simulink model "sphere_6SUR_mech"  (R2017a)
settings: Solver=FixedStepAuto  StartTime=0.0  StopTime=100  FixedStep=0.001  RelTol=1e-2  EnableMultiTasking=on
undefined symbols (not defined in the file): m, rad, s
libraries: mblibv1 x69, simulink x3, instrumentlib x1
(part 1 of 2)
settings Model: SimulationMode=accelerator  Creator=ivanp7  LastModifiedBy=ivanp7
settings OptimizationCC: LifeSpan=inf
settings DebuggingCC: AlgebraicLoopMsg=none  SFUnexpectedBacktrackingDiag=warning  SFNoUnconditionalDefaultTransitionDiag=warning  SFExecutionAtInitializationDiag=none
settings GRTTargetCC: TargetLangStandard=C89/C90 (ANSI)  GeneratePreprocessorConditionals=Disable all
settings ConfigComp: CovMetricSettings=dw  CovHtmlReporting=on  CovSaveCumulativeToWorkspaceVar=on  CovSaveSingleToWorkspaceVar=on  CovExternalEMLEnable=off
settings SimMechanicsCC: LastVizWinPosition=[1141 536 560 420]  CamPosition=[4.37083;-0.373326;26.621;]  CamTarget=[4.37083;-0.373326;0;]  CamUpVector=[0;1;0;]  CamHeight=73.1719  VisBackgroundColor=[0.9;0.9;0.95;]  DefaultBodyColor=[1;0;0;]

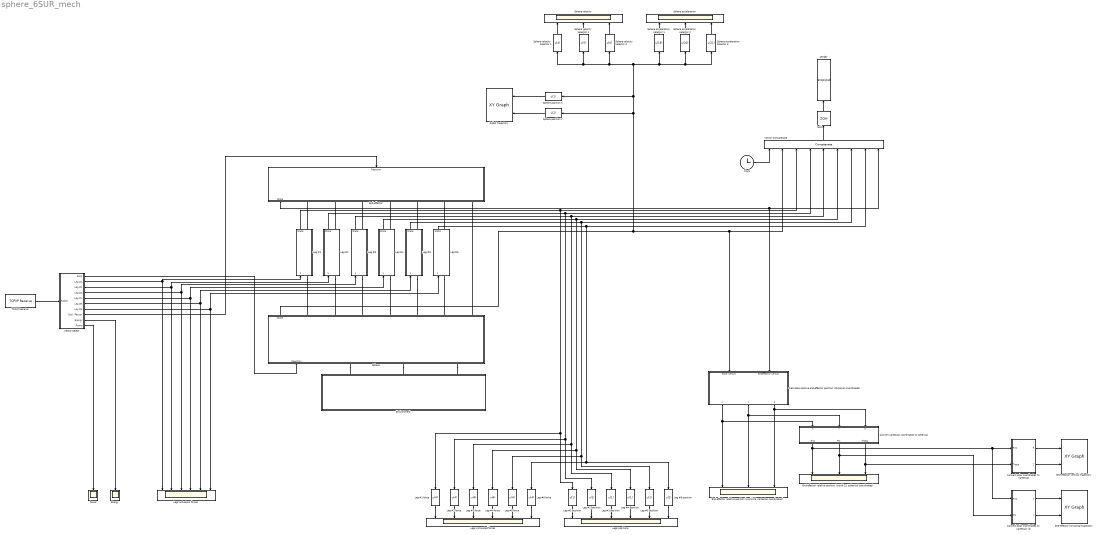
== system sphere_6SUR_mech ==
  Calculate relative end-effector position (cartesian coordinates) : Subsystem
  Convert cartesian coordinates to spherical : Subsystem
  Convert polar coordinates to cartesian : Subsystem
  Convert polar coordinates to cartesian (2) : Subsystem
  End-effector : Subsystem  mask{endeffector_radius=0.25, endeffector_mass=1, endeffector_inertia_coef=2/5}
      mask prompts: endeffector_radius "End-effector radius, m"; endeffector_mass "End-effector mass, kg"; endeffector_inertia_coef "End-effector inertia coefficient"
  End-effector horizontal trajectory : simulink/Sinks/XY Graph  xmin=-1  xmax=1  ymin=-1  ymax=1  st=-1
  "End-effector relative position (world CS, cartesian coordinates)" : Scope  NumInputPorts=3
  "End-effector relative position (world CS, spherical coordinates)" : Scope  NumInputPorts=3
  End-effector vertical trajectory : simulink/Sinks/XY Graph  xmin=0  xmax=1  ymin=-1  ymax=1  st=-1
  Energy : Scope
  Environment : Subsystem  mask{sphere_radius=1, initial_velocity_x=0, initial_velocity_y=0}
      mask prompts: sphere_radius "Sphere radius, m"; initial_velocity_x "Initial velocity (x-axis), m/s"; initial_velocity_y "Initial velocity (y-axis), m/s"
  Leg #1 : Subsystem  mask{ru_mass=0.005, us_mass=0.005, r_axis=[0.505879 -0.310617 0.804738], u_axis1=[0.505879 -0.310617 0.804738], u_axis2=[0.533176 -0.620769 -0.574777], r_coord=[0.12647 -0.0776543 0.201184], u_coord=[-0.382099 -0.61753 0.3125], s_coord=[0 0 1]}
      mask prompts: ru_mass "R-U chain mass, kg"; us_mass "U-S chain mass, kg"; r_axis "R joint axis"; u_axis1 "U joint axis 1"; u_axis2 "U joint axis 2"; r_coord "R joint coordinates"; u_coord "U joint coordinates"; s_coord "S joint coordinates"
  Leg #1 force : Fcn  Expr=u(4)
  Leg #1 position : Fcn  Expr=u(1)
  Leg #2 : Subsystem  mask{ru_mass=0.005, us_mass=0.005, r_axis=[-0.505879 0.310617 -0.804738], u_axis1=[-0.505879 0.310617 -0.804738], u_axis2=[-0.533176 0.620769 0.574777], r_coord=[-0.12647 0.0776543 -0.201184], u_coord=[0.382099 0.61753 -0.3125], s_coord=[0 0 -1]}
      mask prompts: ru_mass "R-U chain mass, kg"; us_mass "U-S chain mass, kg"; r_axis "R joint axis"; u_axis1 "U joint axis 1"; u_axis2 "U joint axis 2"; r_coord "R joint coordinates"; u_coord "U joint coordinates"; s_coord "S joint coordinates"
  Leg #2 force : Fcn  Expr=u(4)
  Leg #2 position : Fcn  Expr=u(1)
  Leg #3 : Subsystem  mask{ru_mass=0.005, us_mass=0.005, r_axis=[0.804738 0.505879 -0.310617], u_axis1=[0.804738 0.505879 -0.310617], u_axis2=[-0.574777 0.533176 -0.620769], r_coord=[0.201184 0.12647 -0.0776543], u_coord=[0.3125 -0.382099 -0.61753], s_coord=[1 0 0]}
      mask prompts: ru_mass "R-U chain mass, kg"; us_mass "U-S chain mass, kg"; r_axis "R joint axis"; u_axis1 "U joint axis 1"; u_axis2 "U joint axis 2"; r_coord "R joint coordinates"; u_coord "U joint coordinates"; s_coord "S joint coordinates"
  Leg #3 force : Fcn  Expr=u(4)
  Leg #3 position : Fcn  Expr=u(1)
  Leg #4 : Subsystem  mask{ru_mass=0.005, us_mass=0.005, r_axis=[-0.804738 -0.505879 0.310617], u_axis1=[-0.804738 -0.505879 0.310617], u_axis2=[0.574777 -0.533176 0.620769], r_coord=[-0.201184 -0.12647 0.0776543], u_coord=[-0.3125 0.382099 0.61753], s_coord=[-1 0 0]}
      mask prompts: ru_mass "R-U chain mass, kg"; us_mass "U-S chain mass, kg"; r_axis "R joint axis"; u_axis1 "U joint axis 1"; u_axis2 "U joint axis 2"; r_coord "R joint coordinates"; u_coord "U joint coordinates"; s_coord "S joint coordinates"
  Leg #4 force : Fcn  Expr=u(4)
  Leg #4 position : Fcn  Expr=u(1)
  Leg #5 : Subsystem  mask{ru_mass=0.005, us_mass=0.005, r_axis=[-0.310617 0.804738 0.505879], u_axis1=[-0.310617 0.804738 0.505879], u_axis2=[-0.620769 -0.574777 0.533176], r_coord=[-0.0776543 0.201184 0.12647], u_coord=[-0.61753 0.3125 -0.382099], s_coord=[0 1 0]}
      mask prompts: ru_mass "R-U chain mass, kg"; us_mass "U-S chain mass, kg"; r_axis "R joint axis"; u_axis1 "U joint axis 1"; u_axis2 "U joint axis 2"; r_coord "R joint coordinates"; u_coord "U joint coordinates"; s_coord "S joint coordinates"
  Leg #5 force : Fcn  Expr=u(4)
  Leg #5 position : Fcn  Expr=u(1)
  Leg #6 : Subsystem  mask{ru_mass=0.005, us_mass=0.005, r_axis=[0.310617 -0.804738 -0.505879], u_axis1=[0.310617 -0.804738 -0.505879], u_axis2=[0.620769 0.574777 -0.533176], r_coord=[0.0776543 -0.201184 -0.12647], u_coord=[0.61753 -0.3125 0.382099], s_coord=[0 -1 0]}
      mask prompts: ru_mass "R-U chain mass, kg"; us_mass "U-S chain mass, kg"; r_axis "R joint axis"; u_axis1 "U joint axis 1"; u_axis2 "U joint axis 2"; r_coord "R joint coordinates"; u_coord "U joint coordinates"; s_coord "S joint coordinates"
  Leg #6 force : Fcn  Expr=u(4)
  Leg #6 position : Fcn  Expr=u(1)
  Legs actuators forces : Scope  NumInputPorts=6
  Legs computed forces : Scope  NumInputPorts=6
  Legs positions : Scope  NumInputPorts=6
  Power : Scope
  Robot trajectory : simulink/Sinks/XY Graph  xmin=-100  xmax=100  ymin=-100  ymax=100  st=-1
  Sphere : Subsystem  mask{sphere_radius=1, sphere_mass=0.1, sphere_inertia_coef=2/3}
      mask prompts: sphere_radius "Sphere radius, m"; sphere_mass "Sphere mass, kg"; sphere_inertia_coef "Sphere inertia coefficient, m"
  Sphere acceleration selector 1 : Fcn  Expr=u(19)
  Sphere acceleration selector 2 : Fcn  Expr=u(20)
  Sphere acceleration selector 3 : Fcn  Expr=u(21)
  Sphere velocity selector 1 : Fcn  Expr=u(4)
  Sphere velocity selector 2 : Fcn  Expr=u(5)
  Sphere velocity selector 3 : Fcn  Expr=u(6)
  Sphere acceleration : Scope  NumInputPorts=3
  Sphere position X : Fcn  Expr=u(1)
  Sphere position Y : Fcn  Expr=u(2)
  Sphere velocity : Scope  NumInputPorts=3
  TCP/IP Receive : instrumentlib/TCP//IP Receive  Priority=1  Host=localhost  Port=61111  DataSize="[1  20]"  EnableBlockingMode=on  Timeout=1  SampleTime=0.001  DataType=double  ByteOrder=LittleEndian
      settings: SourceProductName=Instrument Control Toolbox
  Vector Concatenate : Concatenate  NumInputs=9
  Vector Select : Subsystem
  clock : Clock
      settings: Decimation=1000
  hold : ZeroOrderHold  SampleTime=-1
  sender : M-S-Function  Priority=2  DialogController=instrumentcreatedialog  FunctionName=stcpipsb  Parameters=Host, Port, EnableBlockingMode, Timeout, ByteOrder  DisplayMFileStacktrace=off  mask(TCP/IP Send){Host=localhost, Port=61112, EnableBlockingMode=on, Timeout=1, ByteOrder=LittleEndian}
      mask prompts: Port "Remote Port:"; EnableBlockingMode "Enable blocking mode"; ByteOrder "Byte order:"
      mask help: Send data over TCP/IP network to a specified remote machine.
      mask init:
      | [str port] = instrumentslgate('privateslgetdisplaystring', EnableBlockingMode);
      mask Help: eval('helpview(fullfile(docroot, ''toolbox'', ''instrument'', ''instrument.map''), ''ICT_tcpipsend_Block'')');
      mask TypeOptions ByteOrder: BigEndian | LittleEndian
      mask Display:
      | disp(str);
      | port_label('input',port(1).id,port(1).label);
  wires:
  Leg #1/1(State) -> Vector Concatenate/3, Leg #1 force/1, Leg #1 position/1
  Leg #2/1(State) -> Leg #2 force/1, Leg #2 position/1, Vector Concatenate/4
  Leg #3/1(State) -> Vector Concatenate/5, Leg #3 force/1, Leg #3 position/1
  End-effector/1(State) -> Calculate relative end-effector position (cartesian coordinates)/2(Endeffector sensor), Vector Concatenate/9
  Leg #1 position/1 -> Legs positions/1
  Leg #2 position/1 -> Legs positions/2
  Leg #3 position/1 -> Legs positions/3
  Vector Select/4(Leg #3) -> Leg #3/1(Reaction), Legs actuators forces/3
  Vector Select/2(Leg #1) -> Legs actuators forces/1, Leg #1/1(Reaction)
  Vector Select/3(Leg #2) -> Leg #2/1(Reaction), Legs actuators forces/2
  Vector Select/8(End effector) -> End-effector/1(Reaction)
  Vector Select/1(Body) -> Sphere/1(Reaction)
  Sphere velocity selector 3/1 -> Sphere velocity/3
  Sphere acceleration selector 1/1 -> Sphere acceleration/1
  Sphere acceleration selector 2/1 -> Sphere acceleration/2
  Sphere acceleration selector 3/1 -> Sphere acceleration/3
  Sphere velocity selector 2/1 -> Sphere velocity/2
  Sphere velocity selector 1/1 -> Sphere velocity/1
  Vector Select/9(Energy) -> Energy/1
  Sphere/1(State) -> Calculate relative end-effector position (cartesian coordinates)/1(Body sensor), Vector Concatenate/2, Sphere position X/1, Sphere velocity selector 2/1, Sphere velocity selector 1/1, Sphere velocity selector 3/1, Sphere acceleration selector 1/1, Sphere acceleration selector 2/1, Sphere acceleration selector 3/1, Sphere position Y/1
  Calculate relative end-effector position (cartesian coordinates)/1(X) -> "End-effector relative position (world CS, cartesian coordinates)"/1, Convert cartesian coordinates to spherical/1(X)
  Calculate relative end-effector position (cartesian coordinates)/2(Y) -> "End-effector relative position (world CS, cartesian coordinates)"/2, Convert cartesian coordinates to spherical/2(Y)
  Calculate relative end-effector position (cartesian coordinates)/3(Z) -> "End-effector relative position (world CS, cartesian coordinates)"/3, Convert cartesian coordinates to spherical/3(Z)
  Convert cartesian coordinates to spherical/1(Rho) -> Convert polar coordinates to cartesian (2)/1(Rho), Convert polar coordinates to cartesian/1(Rho), "End-effector relative position (world CS, spherical coordinates)"/1
  Convert cartesian coordinates to spherical/2(Phi) -> Convert polar coordinates to cartesian (2)/2(Phi), "End-effector relative position (world CS, spherical coordinates)"/2
  Convert cartesian coordinates to spherical/3(Theta) -> Convert polar coordinates to cartesian/2(Theta), "End-effector relative position (world CS, spherical coordinates)"/3
  TCP/IP Receive/1 -> Vector Select/1(Robot)
  hold/1 -> sender/1
  Vector Concatenate/1 -> hold/1
  clock/1 -> Vector Concatenate/1
  Leg #2 force/1 -> Legs computed forces/2
  Leg #1 force/1 -> Legs computed forces/1
  Leg #3 force/1 -> Legs computed forces/3
  Vector Select/10(Power) -> Power/1
  Sphere position X/1 -> Robot trajectory/1
  Sphere position Y/1 -> Robot trajectory/2
  Convert polar coordinates to cartesian/1(R) -> End-effector vertical trajectory/1
  Convert polar coordinates to cartesian/2(Z) -> End-effector vertical trajectory/2
  Convert polar coordinates to cartesian (2)/2(Y) -> End-effector horizontal trajectory/2
  Convert polar coordinates to cartesian (2)/1(X) -> End-effector horizontal trajectory/1
  Vector Select/5(Leg #4) -> Leg #4/1(Reaction), Legs actuators forces/4
  Vector Select/6(Leg #5) -> Leg #5/1(Reaction), Legs actuators forces/5
  Vector Select/7(Leg #6) -> Leg #6/1(Reaction), Legs actuators forces/6
  Leg #4/1(State) -> Leg #4 position/1, Leg #4 force/1, Vector Concatenate/6
  Leg #5/1(State) -> Vector Concatenate/7, Leg #5 position/1, Leg #5 force/1
  Leg #6/1(State) -> Vector Concatenate/8, Leg #6 position/1, Leg #6 force/1
  Leg #6 force/1 -> Legs computed forces/6
  Leg #5 force/1 -> Legs computed forces/5
  Leg #4 force/1 -> Legs computed forces/4
  Leg #6 position/1 -> Legs positions/6
  Leg #5 position/1 -> Legs positions/5
  Leg #4 position/1 -> Legs positions/4
  connections:
  Leg #1/LConn1 -- Sphere/RConn1
  Sphere/LConn1 -- Environment/LConn1
  Sphere/LConn2 -- Environment/LConn2
  Sphere/LConn3 -- Environment/LConn3
  Leg #1/RConn1 -- End-effector/RConn1
  End-effector/RConn7 -- Sphere/RConn7
  Leg #2/RConn1 -- End-effector/RConn2
  Leg #3/RConn1 -- End-effector/RConn3
  Leg #2/LConn1 -- Sphere/RConn2
  Leg #5/LConn1 -- Sphere/RConn5
  Leg #3/LConn1 -- Sphere/RConn3
  Leg #6/LConn1 -- Sphere/RConn6
  Leg #4/RConn1 -- End-effector/RConn4
  Leg #4/LConn1 -- Sphere/RConn4
  Leg #5/RConn1 -- End-effector/RConn5
  Leg #6/RConn1 -- End-effector/RConn6

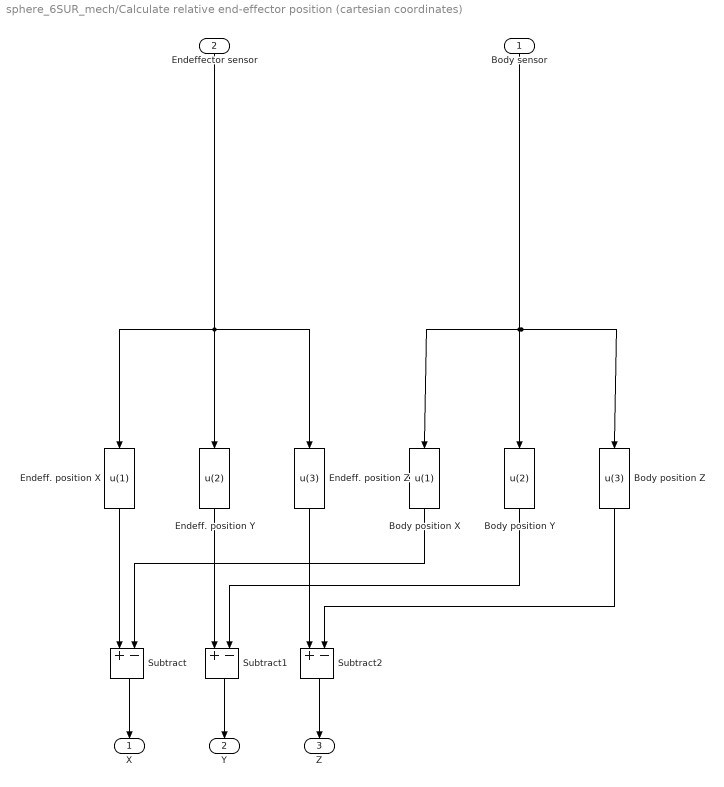
== system sphere_6SUR_mech/Calculate relative end-effector position (cartesian coordinates) ==
  Body sensor : Inport
  Endeffector sensor : Inport  Port=2
  Body position X : Fcn  Expr=u(1)
  Body position Y : Fcn  Expr=u(2)
  Body position Z : Fcn  Expr=u(3)
  Endeff. position X : Fcn  Expr=u(1)
  Endeff. position Y : Fcn  Expr=u(2)
  Endeff. position Z : Fcn  Expr=u(3)
  Subtract : Sum  Inputs=+-
  Subtract1 : Sum  Inputs=+-
  Subtract2 : Sum  Inputs=+-
  X : Outport
  Y : Outport  Port=2
  Z : Outport  Port=3
  wires:
  Body position X/1 -> Subtract/2
  Body position Z/1 -> Subtract2/2
  Subtract/1 -> X/1
  Subtract1/1 -> Y/1
  Endeff. position X/1 -> Subtract/1
  Endeff. position Y/1 -> Subtract1/1
  Endeff. position Z/1 -> Subtract2/1
  Subtract2/1 -> Z/1
  Body sensor/1 -> Body position Z/1, Body position Y/1, Body position X/1
  Body position Y/1 -> Subtract1/2
  Endeffector sensor/1 -> Endeff. position Z/1, Endeff. position X/1, Endeff. position Y/1

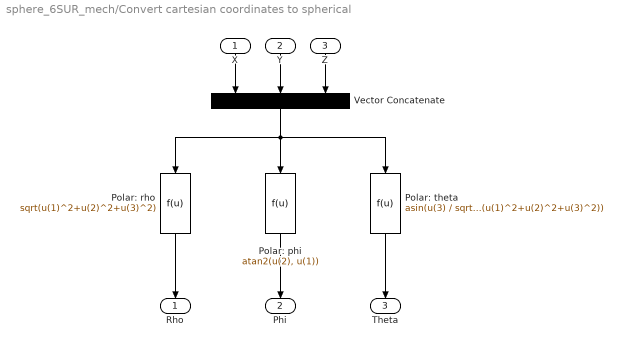
== system sphere_6SUR_mech/Convert cartesian coordinates to spherical ==
  X : Inport
  Y : Inport  Port=2
  Z : Inport  Port=3
  Polar: phi : Fcn  Expr=atan2(u(2), u(1))
  Polar: rho : Fcn  Expr=sqrt(u(1)^2+u(2)^2+u(3)^2)
  Polar: theta : Fcn  Expr=asin(u(3) / sqrt(u(1)^2+u(2)^2+u(3)^2))
  Vector Concatenate : Concatenate  NumInputs=3
  Rho : Outport
  Phi : Outport  Port=2
  Theta : Outport  Port=3
  wires:
  Polar: rho/1 -> Rho/1
  Polar: phi/1 -> Phi/1
  Polar: theta/1 -> Theta/1
  Y/1 -> Vector Concatenate/2
  Z/1 -> Vector Concatenate/3
  X/1 -> Vector Concatenate/1
  Vector Concatenate/1 -> Polar: theta/1, Polar: rho/1, Polar: phi/1

== system sphere_6SUR_mech/Convert polar coordinates to cartesian ==
  Rho : Inport
  Theta : Inport  Port=2
  Cartesian: r : Fcn  Expr=u(1) * cos(u(2))
  Cartesian: z : Fcn  Expr=u(1) * sin(u(2))
  Vector Concatenate : Concatenate
  R : Outport
  Z : Outport  Port=2
  wires:
  Cartesian: r/1 -> R/1
  Cartesian: z/1 -> Z/1
  Theta/1 -> Vector Concatenate/2
  Rho/1 -> Vector Concatenate/1
  Vector Concatenate/1 -> Cartesian: z/1, Cartesian: r/1

== system sphere_6SUR_mech/Convert polar coordinates to cartesian (2) ==
  Rho : Inport
  Phi : Inport  Port=2
  Cartesian: x : Fcn  Expr=u(1) * cos(u(2))
  Cartesian: y : Fcn  Expr=u(1) * sin(u(2))
  Vector Concatenate : Concatenate
  X : Outport
  Y : Outport  Port=2
  wires:
  Cartesian: x/1 -> X/1
  Cartesian: y/1 -> Y/1
  Phi/1 -> Vector Concatenate/2
  Rho/1 -> Vector Concatenate/1
  Vector Concatenate/1 -> Cartesian: y/1, Cartesian: x/1

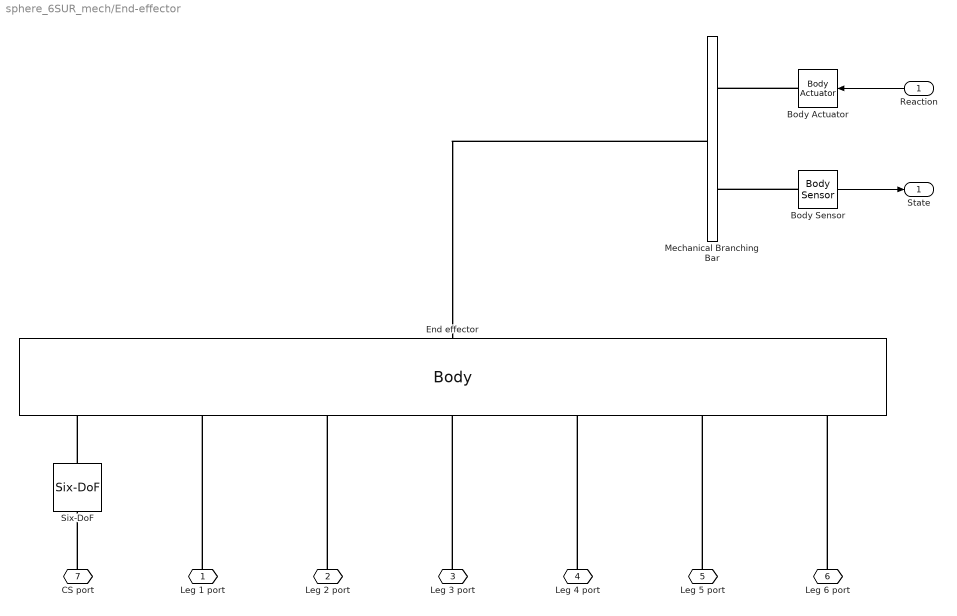
== system sphere_6SUR_mech/End-effector ==
  Reaction : Inport  OutDataTypeStr=double
  Body Actuator : mblibv1/Sensors &  Actuators/Body Actuator  UpdateFromCAD=off  PhysicalDomain=Mechanical  PortType=blob  ActuationStyle=Force  AngleUnits=deg  ArcVelocityUnits=deg/s  ArcAccelerationUnits=deg/s^2  CoordPositionUnits=m  VelocityUnits=m/s  AccelerationUnits=m/s^2  ForceUnits=N  TorqueUnits=N*m  ActiveIO=on  Width=6  DialogClass=MechanicalActuatorBlock  ReferenceFrame=Absolute (World)  Angle=off  CoordPosition=on  Force=on  Torque=on
      settings: SourceProductName=Simscape Multibody  SourceProductBaseCode=MS
  Body Sensor : mblibv1/Sensors &  Actuators/Body Sensor  UpdateFromCAD=off  PhysicalDomain=Mechanical  PortType=blob  Muxed=on  Pose=on  Angle=on  AngleUnits=deg  ArcVelocity=on  ArcVelocityUnits=rad/s  ArcAcceleration=on  ArcAccelerationUnits=rad/s^2  CoordPosition=on  CoordPositionUnits=m  Velocity=on  VelocityUnits=m/s  Acceleration=on  AccelerationUnits=m/s^2  Quaternion=on  QuaternionDT=off  QuaternionDDT=off  QuaternionUnits=off  OutputVector=[1]  ActiveIO=on  Width=24  DialogClass=MechanicalSensorBlock  ReferenceFrame=Absolute (World)
      settings: SourceProductName=Simscape Multibody  SourceProductBaseCode=MS
  End effector : mblibv1/Bodies/Body  LConnTagsString=CS7  RConnTagsString=CG|CS1|CS2|CS3|CS4|CS5|CS6  UpdateFromCAD=off  DialogClass=MechanicalBodyBlock  Mass=endeffector_mass  MassUnits=kg  InertiaUnits=kg*m^2  Inertia=endeffector_inertia_coef*endeffector_mass*endeffector_radius^2*eye(3)  Shape=Cylinder  ShapeDims=[1 1]  ShapeUnits=m  ShapeUse=false  Density=1  DensityUnits=kg/m^3  DensityUse=false  GraphicsMode=CONVHULL  BodyColorSelMode=MACHINE_DEFAULT  BodyColor=[1 0 0]  AttachedToCS=CG  CG=Right$CG$[0;0;0]$World$World$m$[0 0 0]$Euler X-Y-Z$deg$Adjoining$true$none  WorkingFrames=Right$CS1$[0;0;0]$Adjoining$Adjoining$m$[0 0 0]$Euler X-Y-Z$deg$CG$true$none#Right$CS2$[0;0;0]$Adjoining$Adjoining$m$[0 0 0]$Euler X-Y-Z$deg$CG$true$none#Right$CS3$[0;0;0]$Adjoining$Adjoining$m$[0 0 0]$Euler X-Y-Z$deg$CG$true$none#Right$CS4$[0;0;0]$Adjoining$Adjoining$m$[0 0 0]$Euler X-Y-Z$deg$CG$true$none#Right$CS5$[0;0;0]$Adjoining$Adjoining$m$[0 0 0]$Euler X-Y-Z$deg$CG$true$none#Right$CS6$[0;0;0]$Adjoining$Adjoining$m$[0 0 0]$Euler X-Y-Z$deg$CG$true$none#Left$CS7$[0;0;0]$World$World$m$[0 0 0]$Euler X-Y-Z$deg$CG$true$none  CGPos=[0;0;0]  CGRot=[0 0 0]  CS0Pos=[]  CS0Rot=[]  CS1Pos=[0;0;0]  CS1Rot=[0 0 0]  CS2Pos=[0;0;0]  CS2Rot=[0 0 0]  CS3Pos=[0;0;0]  CS3Rot=[0 0 0]  CS4Pos=[0;0;0]  CS4Rot=[0 0 0]  CS5Pos=[0;0;0]  CS5Rot=[0 0 0]  CS6Pos=[0;0;0]  CS6Rot=[0 0 0]  CS7Pos=[0;0;0]  CS7Rot=[0 0 0]  CS8Pos=[]  CS8Rot=[]  CS9Pos=[]  CS9Rot=[]  CS10Pos=[]  CS10Rot=[]  CS11Pos=[]  CS11Rot=[]  CS12Pos=[]  CS12Rot=[]  CS13Pos=[]  CS13Rot=[]  CS14Pos=[]  CS14Rot=[]  CS15Pos=[]  CS15Rot=[]  CS16Pos=[]  CS16Rot=[]  CS17Pos=[]  CS17Rot=[]  CS18Pos=[]  CS18Rot=[]  CS19Pos=[]  CS19Rot=[]  CS20Pos=[]  CS20Rot=[]
      settings: SourceProductName=Simscape Multibody  SourceProductBaseCode=MS
  Mechanical Branching Bar : mblibv1/Utilities/Mechanical Branching Bar  LConnTagsString=_newl0  RConnTagsString=SA0|SA1  UpdateFromCAD=off  DialogClass=MechanicalBranchingBarBlock  NumSAPorts=2
      settings: SourceProductName=Simscape Multibody  SourceProductBaseCode=MS
  Six-DoF : mblibv1/Joints/Six-DoF  LConnTagsString=__newl0  RConnTagsString=__newr0  UpdateFromCAD=off  NumSAPorts=0  CutJoint=off  MarkAsCut=off  Primitives=prismatic_prismatic  PrimitiveProps=P1$WORLD$[1 0 0]$prismatic#P2$WORLD$[0 1 0]$prismatic#P3$WORLD$[0 0 1]$prismatic#S$WORLD$[0 0 0]$spherical  DialogClass=JointBlock  P1Axis=[1 0 0]  P2Axis=[0 1 0]  P3Axis=[0 0 1]  SAxis=[0 0 0]
      settings: SourceProductName=Simscape Multibody  SourceProductBaseCode=MS
  Leg 1 port : PMIOPort  Port=1  Side=Right
  Leg 2 port : PMIOPort  Port=2  Side=Right
  Leg 3 port : PMIOPort  Port=3  Side=Right
  Leg 4 port : PMIOPort  Port=4  Side=Right
  Leg 5 port : PMIOPort  Port=5  Side=Right
  Leg 6 port : PMIOPort  Port=6  Side=Right
  CS port : PMIOPort  Port=7  Side=Right
  State : Outport  OutDataTypeStr=double
  wires:
  Reaction/1 -> Body Actuator/1
  Body Sensor/1 -> State/1
  connections:
  Mechanical Branching Bar/LConn1 -- End effector/LConn1
  Body Actuator/RConn1 -- Mechanical Branching Bar/RConn1
  Six-DoF/RConn1 -- End effector/RConn1
  Body Sensor/LConn1 -- Mechanical Branching Bar/RConn2
  CS port/RConn1 -- Six-DoF/LConn1
  Leg 2 port/RConn1 -- End effector/RConn3
  Leg 1 port/RConn1 -- End effector/RConn2
  Leg 3 port/RConn1 -- End effector/RConn4
  Leg 6 port/RConn1 -- End effector/RConn7
  Leg 5 port/RConn1 -- End effector/RConn6
  Leg 4 port/RConn1 -- End effector/RConn5

== system sphere_6SUR_mech/Environment ==
  Custom Joint : mblibv1/Joints/Custom Joint  LConnTagsString=__newl0|SA1  RConnTagsString=__newr0  UpdateFromCAD=off  NumSAPorts=1  CutJoint=off  MarkAsCut=off  Primitives=prismatic_prismatic_spherical  PrimitiveProps=P1$World$[1 0 0]$prismatic#P2$World$[0 1 0]$prismatic#S$World$[0 0 0]$spherical  DialogClass=JointBlock  R1Axis=[]  R2Axis=[]  R3Axis=[]  P1Axis=[1 0 0]  P2Axis=[0 1 0]  P3Axis=[]  SAxis=[0 0 0]
      settings: SourceProductName=Simscape Multibody  SourceProductBaseCode=MS
  Initial Linear Position : mblibv1/Sensors &  Actuators/Joint Initial Condition  UpdateFromCAD=off  LeftPortType=blob  RightPortType=blob  PhysicalDomain=Mechanical  DialogClass=InitialConditionBlock  InitialConditions=P1$true$0$m$rad$initial_velocity_x$m/s$rad/s#P2$true$0$m$rad$initial_velocity_y$m/s$rad/s#P3$false$0$m$rad$0$m/s$rad/s#R1$false$0$m$rad$0$m/s$rad/s#R2$false$0$m$rad$0$m/s$rad/s#R3$false$0$m$rad$0$m/s$rad/s#S$false$0$m$rad$0$m/s$rad/s  P1PIC=0  P1VIC=initial_velocity_x  P2PIC=0  P2VIC=initial_velocity_y  P3PIC=0  P3VIC=0  R1PIC=0  R1VIC=0  R2PIC=0  R2VIC=0  R3PIC=0  R3VIC=0  SPIC=0  SVIC=0
      settings: SourceProductName=Simscape Multibody  SourceProductBaseCode=MS
  Plane : Subsystem  mask{width=5}
      mask prompts: width "Square width"
  Rolling constraint : Subsystem
  Rolling constraint port 1 : PMIOPort  Port=1  Side=Left
  Rolling constraint port 2 : PMIOPort  Port=2  Side=Left
  Surface : PMIOPort  Port=3  Side=Left
  connections:
  Surface/RConn1 -- Custom Joint/RConn1
  Plane/LConn1 -- Custom Joint/LConn1
  Initial Linear Position/RConn1 -- Custom Joint/LConn2
  Rolling constraint port 2/RConn1 -- Rolling constraint/LConn2
  Rolling constraint port 1/RConn1 -- Rolling constraint/LConn1

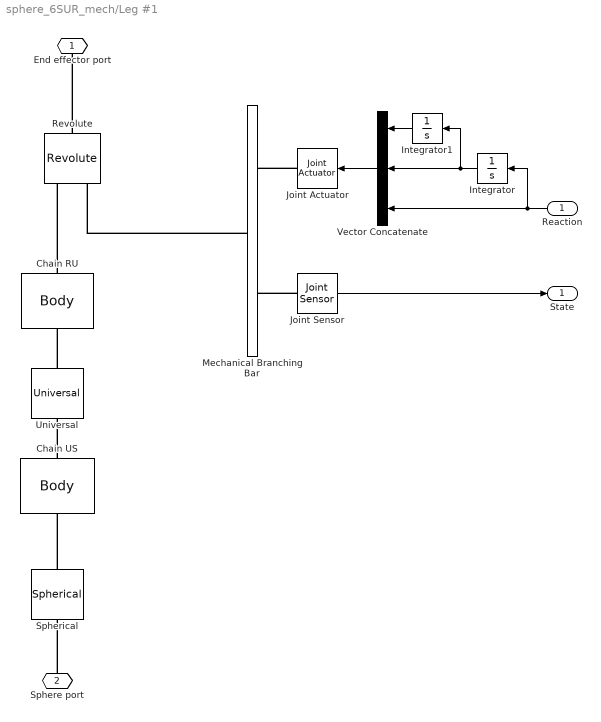
== system sphere_6SUR_mech/Leg #1 ==
  Reaction : Inport
  Chain RU : mblibv1/Bodies/Body  LConnTagsString=CS1  RConnTagsString=CS2  UpdateFromCAD=off  DialogClass=MechanicalBodyBlock  Mass=ru_mass  MassUnits=kg  InertiaUnits=kg*m^2  Inertia=zeros(3)  Shape=Cylinder  ShapeDims=[1 1]  ShapeUnits=m  ShapeUse=false  Density=1  DensityUnits=kg/m^3  DensityUse=false  GraphicsMode=CONVHULL  BodyColorSelMode=COLORPALETTE  BodyColor=[0 1 0]  AttachedToCS=CG  CG=Left$CG$(u_coord+r_coord)/2$World$World$m$[0 0 0]$Euler X-Y-Z$deg$World$false$none  WorkingFrames=Left$CS1$u_coord$World$World$m$[0 0 0]$Euler X-Y-Z$deg$World$true$none#Right$CS2$r_coord$World$World$m$[0 0 0]$Euler X-Y-Z$deg$World$true$none  CGPos=(u_coord+r_coord)/2  CGRot=[0 0 0]  CS0Pos=[]  CS0Rot=[]  CS1Pos=u_coord  CS1Rot=[0 0 0]  CS2Pos=r_coord  CS2Rot=[0 0 0]  CS3Pos=[]  CS3Rot=[]  CS4Pos=[]  CS4Rot=[]  CS5Pos=[]  CS5Rot=[]  CS6Pos=[]  CS6Rot=[]  CS7Pos=[]  CS7Rot=[]  CS8Pos=[]  CS8Rot=[]  CS9Pos=[]  CS9Rot=[]  CS10Pos=[]  CS10Rot=[]  CS11Pos=[]  CS11Rot=[]  CS12Pos=[]  CS12Rot=[]  CS13Pos=[]  CS13Rot=[]  CS14Pos=[]  CS14Rot=[]  CS15Pos=[]  CS15Rot=[]  CS16Pos=[]  CS16Rot=[]  CS17Pos=[]  CS17Rot=[]  CS18Pos=[]  CS18Rot=[]  CS19Pos=[]  CS19Rot=[]  CS20Pos=[]  CS20Rot=[]
      settings: SourceProductName=Simscape Multibody  SourceProductBaseCode=MS
  Chain US : mblibv1/Bodies/Body  LConnTagsString=CS1  RConnTagsString=CS2  UpdateFromCAD=off  DialogClass=MechanicalBodyBlock  Mass=us_mass  MassUnits=kg  InertiaUnits=kg*m^2  Inertia=zeros(3)  Shape=Cylinder  ShapeDims=[1 1]  ShapeUnits=m  ShapeUse=false  Density=1  DensityUnits=kg/m^3  DensityUse=false  GraphicsMode=CONVHULL  BodyColorSelMode=COLORPALETTE  BodyColor=[0 1 0]  AttachedToCS=CG  CG=Left$CG$(s_coord+u_coord)/2$World$World$m$[0 0 0]$Euler X-Y-Z$deg$World$false$none  WorkingFrames=Left$CS1$s_coord$World$World$m$[0 0 0]$Euler X-Y-Z$deg$World$true$none#Right$CS2$u_coord$World$World$m$[0 0 0]$Euler X-Y-Z$deg$World$true$none  CGPos=(s_coord+u_coord)/2  CGRot=[0 0 0]  CS0Pos=[]  CS0Rot=[]  CS1Pos=s_coord  CS1Rot=[0 0 0]  CS2Pos=u_coord  CS2Rot=[0 0 0]  CS3Pos=[]  CS3Rot=[]  CS4Pos=[]  CS4Rot=[]  CS5Pos=[]  CS5Rot=[]  CS6Pos=[]  CS6Rot=[]  CS7Pos=[]  CS7Rot=[]  CS8Pos=[]  CS8Rot=[]  CS9Pos=[]  CS9Rot=[]  CS10Pos=[]  CS10Rot=[]  CS11Pos=[]  CS11Rot=[]  CS12Pos=[]  CS12Rot=[]  CS13Pos=[]  CS13Rot=[]  CS14Pos=[]  CS14Rot=[]  CS15Pos=[]  CS15Rot=[]  CS16Pos=[]  CS16Rot=[]  CS17Pos=[]  CS17Rot=[]  CS18Pos=[]  CS18Rot=[]  CS19Pos=[]  CS19Rot=[]  CS20Pos=[]  CS20Rot=[]
      settings: SourceProductName=Simscape Multibody  SourceProductBaseCode=MS
  Integrator : Integrator
  Integrator1 : Integrator
  Joint Actuator : mblibv1/Sensors &  Actuators/Joint Actuator  UpdateFromCAD=off  PhysicalDomain=Mechanical  PortType=blob  ActuationStyle=Motion  AngleUnits=rad  ArcVelocityUnits=rad/s  ArcAccelerationUnits=rad/s^2  CoordPositionUnits=m  VelocityUnits=m/s  AccelerationUnits=m/s^2  ForceUnits=N  TorqueUnits=N*m  ActiveIO=on  Width=3  DialogClass=MechanicalActuatorBlock  Primitive=R1  ReferenceFrame=Absolute (World)
      settings: SourceProductName=Simscape Multibody  SourceProductBaseCode=MS
  Joint Sensor : mblibv1/Sensors &  Actuators/Joint Sensor  UpdateFromCAD=off  PhysicalDomain=Mechanical  PortType=blob  Muxed=on  Pose=off  Angle=on  AngleUnits=rad  ArcVelocity=on  ArcVelocityUnits=rad/s  ArcAcceleration=on  ArcAccelerationUnits=rad/s^2  CoordPosition=on  CoordPositionUnits=m  Velocity=on  VelocityUnits=m/s  Acceleration=on  AccelerationUnits=m/s^2  Quaternion=on  QuaternionDT=off  QuaternionDDT=off  QuaternionUnits=off  OutputVector=[1]  ActiveIO=on  Width=10  DialogClass=MechanicalSensorBlock  Primitive=R1  Force=on  ForceUnits=N  Torque=on  TorqueUnits=N*m  ReferenceFrame=Absolute (World)  ReactionSensedSide=Base  ReactionReferenceFrame=Local (Body CS)  ReactionForce=on  ReactionForceUnits=N  ReactionMoment=on  ReactionMomentUnits=N*m
      settings: SourceProductName=Simscape Multibody  SourceProductBaseCode=MS
  Mechanical Branching Bar : mblibv1/Utilities/Mechanical Branching Bar  LConnTagsString=_newl0  RConnTagsString=SA0|SA1  UpdateFromCAD=off  DialogClass=MechanicalBranchingBarBlock  NumSAPorts=2
      settings: SourceProductName=Simscape Multibody  SourceProductBaseCode=MS
  Revolute : mblibv1/Joints/Revolute  LConnTagsString=__newl0|SA1  RConnTagsString=__newr0  UpdateFromCAD=off  NumSAPorts=1  CutJoint=off  MarkAsCut=off  Primitives=prismatic  PrimitiveProps=R1$World$r_axis$revolute  DialogClass=JointBlock  R1Axis=r_axis
      settings: SourceProductName=Simscape Multibody  SourceProductBaseCode=MS
  Spherical : mblibv1/Joints/Spherical  LConnTagsString=__newl0  RConnTagsString=__newr0  UpdateFromCAD=off  NumSAPorts=0  CutJoint=off  MarkAsCut=off  Primitives=spherical  PrimitiveProps=S$WORLD$[0 0 0]$spherical  DialogClass=JointBlock  SAxis=[0 0 0]
      settings: SourceProductName=Simscape Multibody  SourceProductBaseCode=MS
  Universal : mblibv1/Joints/Universal  LConnTagsString=__newl0  RConnTagsString=__newr0  UpdateFromCAD=off  NumSAPorts=0  CutJoint=off  MarkAsCut=off  Primitives=prismatic  PrimitiveProps=R1$World$u_axis1$revolute#R2$World$u_axis2$revolute  DialogClass=JointBlock  R1Axis=u_axis1  R2Axis=u_axis2
      settings: SourceProductName=Simscape Multibody  SourceProductBaseCode=MS
  Vector Concatenate : Concatenate  NumInputs=3
  End effector port : PMIOPort  Port=1  Side=Right
  Sphere port : PMIOPort  Port=2  Side=Left
  State : Outport
  wires:
  Joint Sensor/1 -> State/1
  Vector Concatenate/1 -> Joint Actuator/1
  Reaction/1 -> Integrator/1, Vector Concatenate/3
  Integrator/1 -> Integrator1/1, Vector Concatenate/2
  Integrator1/1 -> Vector Concatenate/1
  connections:
  Revolute/RConn1 -- End effector port/RConn1
  Joint Actuator/RConn1 -- Mechanical Branching Bar/RConn1
  Chain RU/RConn1 -- Revolute/LConn1
  Mechanical Branching Bar/LConn1 -- Revolute/LConn2
  Joint Sensor/LConn1 -- Mechanical Branching Bar/RConn2
  Spherical/RConn1 -- Chain US/LConn1
  Universal/RConn1 -- Chain RU/LConn1
  Chain US/RConn1 -- Universal/LConn1
  Sphere port/RConn1 -- Spherical/LConn1

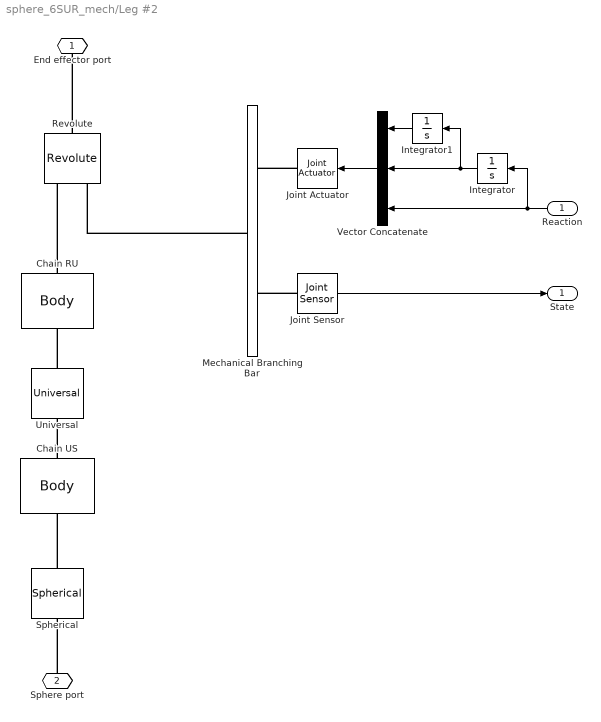
== system sphere_6SUR_mech/Leg #2 ==
  Reaction : Inport
  Chain RU : mblibv1/Bodies/Body  LConnTagsString=CS1  RConnTagsString=CS2  UpdateFromCAD=off  DialogClass=MechanicalBodyBlock  Mass=ru_mass  MassUnits=kg  InertiaUnits=kg*m^2  Inertia=zeros(3)  Shape=Cylinder  ShapeDims=[1 1]  ShapeUnits=m  ShapeUse=false  Density=1  DensityUnits=kg/m^3  DensityUse=false  GraphicsMode=CONVHULL  BodyColorSelMode=COLORPALETTE  BodyColor=[0 1 0]  AttachedToCS=CG  CG=Left$CG$(u_coord+r_coord)/2$World$World$m$[0 0 0]$Euler X-Y-Z$deg$World$false$none  WorkingFrames=Left$CS1$u_coord$World$World$m$[0 0 0]$Euler X-Y-Z$deg$World$true$none#Right$CS2$r_coord$World$World$m$[0 0 0]$Euler X-Y-Z$deg$World$true$none  CGPos=(u_coord+r_coord)/2  CGRot=[0 0 0]  CS0Pos=[]  CS0Rot=[]  CS1Pos=u_coord  CS1Rot=[0 0 0]  CS2Pos=r_coord  CS2Rot=[0 0 0]  CS3Pos=[]  CS3Rot=[]  CS4Pos=[]  CS4Rot=[]  CS5Pos=[]  CS5Rot=[]  CS6Pos=[]  CS6Rot=[]  CS7Pos=[]  CS7Rot=[]  CS8Pos=[]  CS8Rot=[]  CS9Pos=[]  CS9Rot=[]  CS10Pos=[]  CS10Rot=[]  CS11Pos=[]  CS11Rot=[]  CS12Pos=[]  CS12Rot=[]  CS13Pos=[]  CS13Rot=[]  CS14Pos=[]  CS14Rot=[]  CS15Pos=[]  CS15Rot=[]  CS16Pos=[]  CS16Rot=[]  CS17Pos=[]  CS17Rot=[]  CS18Pos=[]  CS18Rot=[]  CS19Pos=[]  CS19Rot=[]  CS20Pos=[]  CS20Rot=[]
      settings: SourceProductName=Simscape Multibody  SourceProductBaseCode=MS
  Chain US : mblibv1/Bodies/Body  LConnTagsString=CS1  RConnTagsString=CS2  UpdateFromCAD=off  DialogClass=MechanicalBodyBlock  Mass=us_mass  MassUnits=kg  InertiaUnits=kg*m^2  Inertia=zeros(3)  Shape=Cylinder  ShapeDims=[1 1]  ShapeUnits=m  ShapeUse=false  Density=1  DensityUnits=kg/m^3  DensityUse=false  GraphicsMode=CONVHULL  BodyColorSelMode=COLORPALETTE  BodyColor=[0 1 0]  AttachedToCS=CG  CG=Left$CG$(s_coord+u_coord)/2$World$World$m$[0 0 0]$Euler X-Y-Z$deg$World$false$none  WorkingFrames=Left$CS1$s_coord$World$World$m$[0 0 0]$Euler X-Y-Z$deg$World$true$none#Right$CS2$u_coord$World$World$m$[0 0 0]$Euler X-Y-Z$deg$World$true$none  CGPos=(s_coord+u_coord)/2  CGRot=[0 0 0]  CS0Pos=[]  CS0Rot=[]  CS1Pos=s_coord  CS1Rot=[0 0 0]  CS2Pos=u_coord  CS2Rot=[0 0 0]  CS3Pos=[]  CS3Rot=[]  CS4Pos=[]  CS4Rot=[]  CS5Pos=[]  CS5Rot=[]  CS6Pos=[]  CS6Rot=[]  CS7Pos=[]  CS7Rot=[]  CS8Pos=[]  CS8Rot=[]  CS9Pos=[]  CS9Rot=[]  CS10Pos=[]  CS10Rot=[]  CS11Pos=[]  CS11Rot=[]  CS12Pos=[]  CS12Rot=[]  CS13Pos=[]  CS13Rot=[]  CS14Pos=[]  CS14Rot=[]  CS15Pos=[]  CS15Rot=[]  CS16Pos=[]  CS16Rot=[]  CS17Pos=[]  CS17Rot=[]  CS18Pos=[]  CS18Rot=[]  CS19Pos=[]  CS19Rot=[]  CS20Pos=[]  CS20Rot=[]
      settings: SourceProductName=Simscape Multibody  SourceProductBaseCode=MS
  Integrator : Integrator
  Integrator1 : Integrator
  Joint Actuator : mblibv1/Sensors &  Actuators/Joint Actuator  UpdateFromCAD=off  PhysicalDomain=Mechanical  PortType=blob  ActuationStyle=Motion  AngleUnits=rad  ArcVelocityUnits=rad/s  ArcAccelerationUnits=rad/s^2  CoordPositionUnits=m  VelocityUnits=m/s  AccelerationUnits=m/s^2  ForceUnits=N  TorqueUnits=N*m  ActiveIO=on  Width=3  DialogClass=MechanicalActuatorBlock  Primitive=R1  ReferenceFrame=Absolute (World)
      settings: SourceProductName=Simscape Multibody  SourceProductBaseCode=MS
  Joint Sensor : mblibv1/Sensors &  Actuators/Joint Sensor  UpdateFromCAD=off  PhysicalDomain=Mechanical  PortType=blob  Muxed=on  Pose=off  Angle=on  AngleUnits=rad  ArcVelocity=on  ArcVelocityUnits=rad/s  ArcAcceleration=on  ArcAccelerationUnits=rad/s^2  CoordPosition=on  CoordPositionUnits=m  Velocity=on  VelocityUnits=m/s  Acceleration=on  AccelerationUnits=m/s^2  Quaternion=on  QuaternionDT=off  QuaternionDDT=off  QuaternionUnits=off  OutputVector=[1]  ActiveIO=on  Width=10  DialogClass=MechanicalSensorBlock  Primitive=R1  Force=on  ForceUnits=N  Torque=on  TorqueUnits=N*m  ReferenceFrame=Absolute (World)  ReactionSensedSide=Base  ReactionReferenceFrame=Local (Body CS)  ReactionForce=on  ReactionForceUnits=N  ReactionMoment=on  ReactionMomentUnits=N*m
      settings: SourceProductName=Simscape Multibody  SourceProductBaseCode=MS
  Mechanical Branching Bar : mblibv1/Utilities/Mechanical Branching Bar  LConnTagsString=_newl0  RConnTagsString=SA0|SA1  UpdateFromCAD=off  DialogClass=MechanicalBranchingBarBlock  NumSAPorts=2
      settings: SourceProductName=Simscape Multibody  SourceProductBaseCode=MS
  Revolute : mblibv1/Joints/Revolute  LConnTagsString=__newl0|SA1  RConnTagsString=__newr0  UpdateFromCAD=off  NumSAPorts=1  CutJoint=off  MarkAsCut=off  Primitives=prismatic  PrimitiveProps=R1$World$r_axis$revolute  DialogClass=JointBlock  R1Axis=r_axis
      settings: SourceProductName=Simscape Multibody  SourceProductBaseCode=MS
  Spherical : mblibv1/Joints/Spherical  LConnTagsString=__newl0  RConnTagsString=__newr0  UpdateFromCAD=off  NumSAPorts=0  CutJoint=off  MarkAsCut=off  Primitives=spherical  PrimitiveProps=S$WORLD$[0 0 0]$spherical  DialogClass=JointBlock  SAxis=[0 0 0]
      settings: SourceProductName=Simscape Multibody  SourceProductBaseCode=MS
  Universal : mblibv1/Joints/Universal  LConnTagsString=__newl0  RConnTagsString=__newr0  UpdateFromCAD=off  NumSAPorts=0  CutJoint=off  MarkAsCut=off  Primitives=prismatic  PrimitiveProps=R1$World$u_axis1$revolute#R2$World$u_axis2$revolute  DialogClass=JointBlock  R1Axis=u_axis1  R2Axis=u_axis2
      settings: SourceProductName=Simscape Multibody  SourceProductBaseCode=MS
  Vector Concatenate : Concatenate  NumInputs=3
  End effector port : PMIOPort  Port=1  Side=Right
  Sphere port : PMIOPort  Port=2  Side=Left
  State : Outport
  wires:
  Joint Sensor/1 -> State/1
  Vector Concatenate/1 -> Joint Actuator/1
  Reaction/1 -> Integrator/1, Vector Concatenate/3
  Integrator/1 -> Integrator1/1, Vector Concatenate/2
  Integrator1/1 -> Vector Concatenate/1
  connections:
  Revolute/RConn1 -- End effector port/RConn1
  Joint Actuator/RConn1 -- Mechanical Branching Bar/RConn1
  Chain RU/RConn1 -- Revolute/LConn1
  Mechanical Branching Bar/LConn1 -- Revolute/LConn2
  Joint Sensor/LConn1 -- Mechanical Branching Bar/RConn2
  Spherical/RConn1 -- Chain US/LConn1
  Universal/RConn1 -- Chain RU/LConn1
  Chain US/RConn1 -- Universal/LConn1
  Sphere port/RConn1 -- Spherical/LConn1

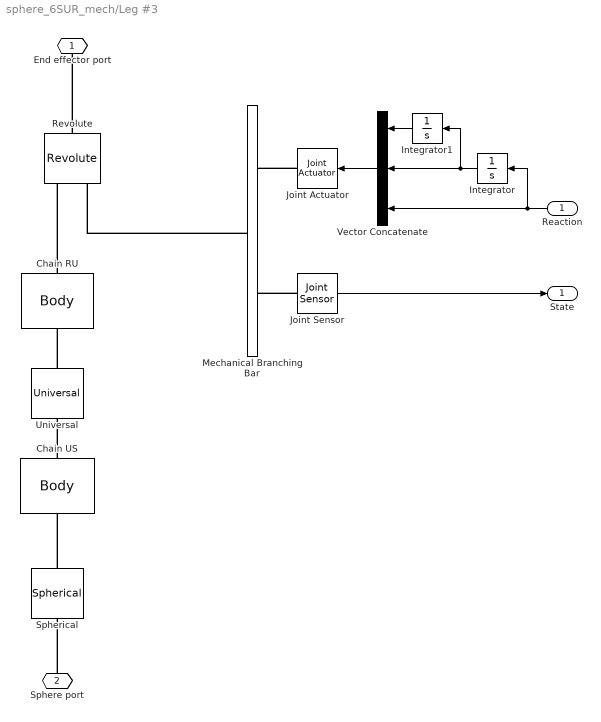
== system sphere_6SUR_mech/Leg #3 ==
  Reaction : Inport
  Chain RU : mblibv1/Bodies/Body  LConnTagsString=CS1  RConnTagsString=CS2  UpdateFromCAD=off  DialogClass=MechanicalBodyBlock  Mass=ru_mass  MassUnits=kg  InertiaUnits=kg*m^2  Inertia=zeros(3)  Shape=Cylinder  ShapeDims=[1 1]  ShapeUnits=m  ShapeUse=false  Density=1  DensityUnits=kg/m^3  DensityUse=false  GraphicsMode=CONVHULL  BodyColorSelMode=COLORPALETTE  BodyColor=[0 1 0]  AttachedToCS=CG  CG=Left$CG$(u_coord+r_coord)/2$World$World$m$[0 0 0]$Euler X-Y-Z$deg$World$false$none  WorkingFrames=Left$CS1$u_coord$World$World$m$[0 0 0]$Euler X-Y-Z$deg$World$true$none#Right$CS2$r_coord$World$World$m$[0 0 0]$Euler X-Y-Z$deg$World$true$none  CGPos=(u_coord+r_coord)/2  CGRot=[0 0 0]  CS0Pos=[]  CS0Rot=[]  CS1Pos=u_coord  CS1Rot=[0 0 0]  CS2Pos=r_coord  CS2Rot=[0 0 0]  CS3Pos=[]  CS3Rot=[]  CS4Pos=[]  CS4Rot=[]  CS5Pos=[]  CS5Rot=[]  CS6Pos=[]  CS6Rot=[]  CS7Pos=[]  CS7Rot=[]  CS8Pos=[]  CS8Rot=[]  CS9Pos=[]  CS9Rot=[]  CS10Pos=[]  CS10Rot=[]  CS11Pos=[]  CS11Rot=[]  CS12Pos=[]  CS12Rot=[]  CS13Pos=[]  CS13Rot=[]  CS14Pos=[]  CS14Rot=[]  CS15Pos=[]  CS15Rot=[]  CS16Pos=[]  CS16Rot=[]  CS17Pos=[]  CS17Rot=[]  CS18Pos=[]  CS18Rot=[]  CS19Pos=[]  CS19Rot=[]  CS20Pos=[]  CS20Rot=[]
      settings: SourceProductName=Simscape Multibody  SourceProductBaseCode=MS
  Chain US : mblibv1/Bodies/Body  LConnTagsString=CS1  RConnTagsString=CS2  UpdateFromCAD=off  DialogClass=MechanicalBodyBlock  Mass=us_mass  MassUnits=kg  InertiaUnits=kg*m^2  Inertia=zeros(3)  Shape=Cylinder  ShapeDims=[1 1]  ShapeUnits=m  ShapeUse=false  Density=1  DensityUnits=kg/m^3  DensityUse=false  GraphicsMode=CONVHULL  BodyColorSelMode=COLORPALETTE  BodyColor=[0 1 0]  AttachedToCS=CG  CG=Left$CG$(s_coord+u_coord)/2$World$World$m$[0 0 0]$Euler X-Y-Z$deg$World$false$none  WorkingFrames=Left$CS1$s_coord$World$World$m$[0 0 0]$Euler X-Y-Z$deg$World$true$none#Right$CS2$u_coord$World$World$m$[0 0 0]$Euler X-Y-Z$deg$World$true$none  CGPos=(s_coord+u_coord)/2  CGRot=[0 0 0]  CS0Pos=[]  CS0Rot=[]  CS1Pos=s_coord  CS1Rot=[0 0 0]  CS2Pos=u_coord  CS2Rot=[0 0 0]  CS3Pos=[]  CS3Rot=[]  CS4Pos=[]  CS4Rot=[]  CS5Pos=[]  CS5Rot=[]  CS6Pos=[]  CS6Rot=[]  CS7Pos=[]  CS7Rot=[]  CS8Pos=[]  CS8Rot=[]  CS9Pos=[]  CS9Rot=[]  CS10Pos=[]  CS10Rot=[]  CS11Pos=[]  CS11Rot=[]  CS12Pos=[]  CS12Rot=[]  CS13Pos=[]  CS13Rot=[]  CS14Pos=[]  CS14Rot=[]  CS15Pos=[]  CS15Rot=[]  CS16Pos=[]  CS16Rot=[]  CS17Pos=[]  CS17Rot=[]  CS18Pos=[]  CS18Rot=[]  CS19Pos=[]  CS19Rot=[]  CS20Pos=[]  CS20Rot=[]
      settings: SourceProductName=Simscape Multibody  SourceProductBaseCode=MS
  Integrator : Integrator
  Integrator1 : Integrator
  Joint Actuator : mblibv1/Sensors &  Actuators/Joint Actuator  UpdateFromCAD=off  PhysicalDomain=Mechanical  PortType=blob  ActuationStyle=Motion  AngleUnits=rad  ArcVelocityUnits=rad/s  ArcAccelerationUnits=rad/s^2  CoordPositionUnits=m  VelocityUnits=m/s  AccelerationUnits=m/s^2  ForceUnits=N  TorqueUnits=N*m  ActiveIO=on  Width=3  DialogClass=MechanicalActuatorBlock  Primitive=R1  ReferenceFrame=Absolute (World)
      settings: SourceProductName=Simscape Multibody  SourceProductBaseCode=MS
  Joint Sensor : mblibv1/Sensors &  Actuators/Joint Sensor  UpdateFromCAD=off  PhysicalDomain=Mechanical  PortType=blob  Muxed=on  Pose=off  Angle=on  AngleUnits=rad  ArcVelocity=on  ArcVelocityUnits=rad/s  ArcAcceleration=on  ArcAccelerationUnits=rad/s^2  CoordPosition=on  CoordPositionUnits=m  Velocity=on  VelocityUnits=m/s  Acceleration=on  AccelerationUnits=m/s^2  Quaternion=on  QuaternionDT=off  QuaternionDDT=off  QuaternionUnits=off  OutputVector=[1]  ActiveIO=on  Width=10  DialogClass=MechanicalSensorBlock  Primitive=R1  Force=on  ForceUnits=N  Torque=on  TorqueUnits=N*m  ReferenceFrame=Absolute (World)  ReactionSensedSide=Base  ReactionReferenceFrame=Local (Body CS)  ReactionForce=on  ReactionForceUnits=N  ReactionMoment=on  ReactionMomentUnits=N*m
      settings: SourceProductName=Simscape Multibody  SourceProductBaseCode=MS
  Mechanical Branching Bar : mblibv1/Utilities/Mechanical Branching Bar  LConnTagsString=_newl0  RConnTagsString=SA0|SA1  UpdateFromCAD=off  DialogClass=MechanicalBranchingBarBlock  NumSAPorts=2
      settings: SourceProductName=Simscape Multibody  SourceProductBaseCode=MS
  Revolute : mblibv1/Joints/Revolute  LConnTagsString=__newl0|SA1  RConnTagsString=__newr0  UpdateFromCAD=off  NumSAPorts=1  CutJoint=off  MarkAsCut=off  Primitives=prismatic  PrimitiveProps=R1$World$r_axis$revolute  DialogClass=JointBlock  R1Axis=r_axis
      settings: SourceProductName=Simscape Multibody  SourceProductBaseCode=MS
  Spherical : mblibv1/Joints/Spherical  LConnTagsString=__newl0  RConnTagsString=__newr0  UpdateFromCAD=off  NumSAPorts=0  CutJoint=off  MarkAsCut=off  Primitives=spherical  PrimitiveProps=S$WORLD$[0 0 0]$spherical  DialogClass=JointBlock  SAxis=[0 0 0]
      settings: SourceProductName=Simscape Multibody  SourceProductBaseCode=MS
  Universal : mblibv1/Joints/Universal  LConnTagsString=__newl0  RConnTagsString=__newr0  UpdateFromCAD=off  NumSAPorts=0  CutJoint=off  MarkAsCut=off  Primitives=prismatic  PrimitiveProps=R1$World$u_axis1$revolute#R2$World$u_axis2$revolute  DialogClass=JointBlock  R1Axis=u_axis1  R2Axis=u_axis2
      settings: SourceProductName=Simscape Multibody  SourceProductBaseCode=MS
  Vector Concatenate : Concatenate  NumInputs=3
  End effector port : PMIOPort  Port=1  Side=Right
  Sphere port : PMIOPort  Port=2  Side=Left
  State : Outport
  wires:
  Joint Sensor/1 -> State/1
  Vector Concatenate/1 -> Joint Actuator/1
  Reaction/1 -> Integrator/1, Vector Concatenate/3
  Integrator/1 -> Integrator1/1, Vector Concatenate/2
  Integrator1/1 -> Vector Concatenate/1
  connections:
  Revolute/RConn1 -- End effector port/RConn1
  Joint Actuator/RConn1 -- Mechanical Branching Bar/RConn1
  Chain RU/RConn1 -- Revolute/LConn1
  Mechanical Branching Bar/LConn1 -- Revolute/LConn2
  Joint Sensor/LConn1 -- Mechanical Branching Bar/RConn2
  Spherical/RConn1 -- Chain US/LConn1
  Universal/RConn1 -- Chain RU/LConn1
  Chain US/RConn1 -- Universal/LConn1
  Sphere port/RConn1 -- Spherical/LConn1

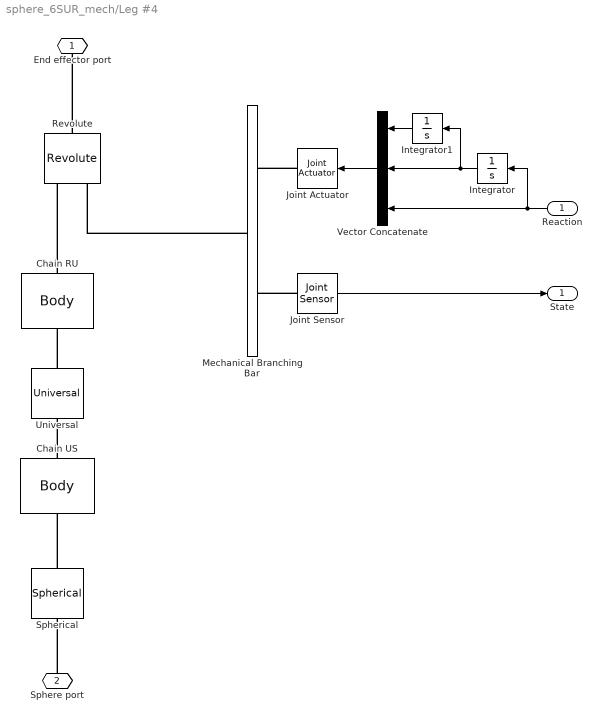
== system sphere_6SUR_mech/Leg #4 ==
  Reaction : Inport
  Chain RU : mblibv1/Bodies/Body  LConnTagsString=CS1  RConnTagsString=CS2  UpdateFromCAD=off  DialogClass=MechanicalBodyBlock  Mass=ru_mass  MassUnits=kg  InertiaUnits=kg*m^2  Inertia=zeros(3)  Shape=Cylinder  ShapeDims=[1 1]  ShapeUnits=m  ShapeUse=false  Density=1  DensityUnits=kg/m^3  DensityUse=false  GraphicsMode=CONVHULL  BodyColorSelMode=COLORPALETTE  BodyColor=[0 1 0]  AttachedToCS=CG  CG=Left$CG$(u_coord+r_coord)/2$World$World$m$[0 0 0]$Euler X-Y-Z$deg$World$false$none  WorkingFrames=Left$CS1$u_coord$World$World$m$[0 0 0]$Euler X-Y-Z$deg$World$true$none#Right$CS2$r_coord$World$World$m$[0 0 0]$Euler X-Y-Z$deg$World$true$none  CGPos=(u_coord+r_coord)/2  CGRot=[0 0 0]  CS0Pos=[]  CS0Rot=[]  CS1Pos=u_coord  CS1Rot=[0 0 0]  CS2Pos=r_coord  CS2Rot=[0 0 0]  CS3Pos=[]  CS3Rot=[]  CS4Pos=[]  CS4Rot=[]  CS5Pos=[]  CS5Rot=[]  CS6Pos=[]  CS6Rot=[]  CS7Pos=[]  CS7Rot=[]  CS8Pos=[]  CS8Rot=[]  CS9Pos=[]  CS9Rot=[]  CS10Pos=[]  CS10Rot=[]  CS11Pos=[]  CS11Rot=[]  CS12Pos=[]  CS12Rot=[]  CS13Pos=[]  CS13Rot=[]  CS14Pos=[]  CS14Rot=[]  CS15Pos=[]  CS15Rot=[]  CS16Pos=[]  CS16Rot=[]  CS17Pos=[]  CS17Rot=[]  CS18Pos=[]  CS18Rot=[]  CS19Pos=[]  CS19Rot=[]  CS20Pos=[]  CS20Rot=[]
      settings: SourceProductName=Simscape Multibody  SourceProductBaseCode=MS
  Chain US : mblibv1/Bodies/Body  LConnTagsString=CS1  RConnTagsString=CS2  UpdateFromCAD=off  DialogClass=MechanicalBodyBlock  Mass=us_mass  MassUnits=kg  InertiaUnits=kg*m^2  Inertia=zeros(3)  Shape=Cylinder  ShapeDims=[1 1]  ShapeUnits=m  ShapeUse=false  Density=1  DensityUnits=kg/m^3  DensityUse=false  GraphicsMode=CONVHULL  BodyColorSelMode=COLORPALETTE  BodyColor=[0 1 0]  AttachedToCS=CG  CG=Left$CG$(s_coord+u_coord)/2$World$World$m$[0 0 0]$Euler X-Y-Z$deg$World$false$none  WorkingFrames=Left$CS1$s_coord$World$World$m$[0 0 0]$Euler X-Y-Z$deg$World$true$none#Right$CS2$u_coord$World$World$m$[0 0 0]$Euler X-Y-Z$deg$World$true$none  CGPos=(s_coord+u_coord)/2  CGRot=[0 0 0]  CS0Pos=[]  CS0Rot=[]  CS1Pos=s_coord  CS1Rot=[0 0 0]  CS2Pos=u_coord  CS2Rot=[0 0 0]  CS3Pos=[]  CS3Rot=[]  CS4Pos=[]  CS4Rot=[]  CS5Pos=[]  CS5Rot=[]  CS6Pos=[]  CS6Rot=[]  CS7Pos=[]  CS7Rot=[]  CS8Pos=[]  CS8Rot=[]  CS9Pos=[]  CS9Rot=[]  CS10Pos=[]  CS10Rot=[]  CS11Pos=[]  CS11Rot=[]  CS12Pos=[]  CS12Rot=[]  CS13Pos=[]  CS13Rot=[]  CS14Pos=[]  CS14Rot=[]  CS15Pos=[]  CS15Rot=[]  CS16Pos=[]  CS16Rot=[]  CS17Pos=[]  CS17Rot=[]  CS18Pos=[]  CS18Rot=[]  CS19Pos=[]  CS19Rot=[]  CS20Pos=[]  CS20Rot=[]
      settings: SourceProductName=Simscape Multibody  SourceProductBaseCode=MS
  Integrator : Integrator
  Integrator1 : Integrator
  Joint Actuator : mblibv1/Sensors &  Actuators/Joint Actuator  UpdateFromCAD=off  PhysicalDomain=Mechanical  PortType=blob  ActuationStyle=Motion  AngleUnits=rad  ArcVelocityUnits=rad/s  ArcAccelerationUnits=rad/s^2  CoordPositionUnits=m  VelocityUnits=m/s  AccelerationUnits=m/s^2  ForceUnits=N  TorqueUnits=N*m  ActiveIO=on  Width=3  DialogClass=MechanicalActuatorBlock  Primitive=R1  ReferenceFrame=Absolute (World)
      settings: SourceProductName=Simscape Multibody  SourceProductBaseCode=MS
  Joint Sensor : mblibv1/Sensors &  Actuators/Joint Sensor  UpdateFromCAD=off  PhysicalDomain=Mechanical  PortType=blob  Muxed=on  Pose=off  Angle=on  AngleUnits=rad  ArcVelocity=on  ArcVelocityUnits=rad/s  ArcAcceleration=on  ArcAccelerationUnits=rad/s^2  CoordPosition=on  CoordPositionUnits=m  Velocity=on  VelocityUnits=m/s  Acceleration=on  AccelerationUnits=m/s^2  Quaternion=on  QuaternionDT=off  QuaternionDDT=off  QuaternionUnits=off  OutputVector=[1]  ActiveIO=on  Width=10  DialogClass=MechanicalSensorBlock  Primitive=R1  Force=on  ForceUnits=N  Torque=on  TorqueUnits=N*m  ReferenceFrame=Absolute (World)  ReactionSensedSide=Base  ReactionReferenceFrame=Local (Body CS)  ReactionForce=on  ReactionForceUnits=N  ReactionMoment=on  ReactionMomentUnits=N*m
      settings: SourceProductName=Simscape Multibody  SourceProductBaseCode=MS
  Mechanical Branching Bar : mblibv1/Utilities/Mechanical Branching Bar  LConnTagsString=_newl0  RConnTagsString=SA0|SA1  UpdateFromCAD=off  DialogClass=MechanicalBranchingBarBlock  NumSAPorts=2
      settings: SourceProductName=Simscape Multibody  SourceProductBaseCode=MS
  Revolute : mblibv1/Joints/Revolute  LConnTagsString=__newl0|SA1  RConnTagsString=__newr0  UpdateFromCAD=off  NumSAPorts=1  CutJoint=off  MarkAsCut=off  Primitives=prismatic  PrimitiveProps=R1$World$r_axis$revolute  DialogClass=JointBlock  R1Axis=r_axis
      settings: SourceProductName=Simscape Multibody  SourceProductBaseCode=MS
  Spherical : mblibv1/Joints/Spherical  LConnTagsString=__newl0  RConnTagsString=__newr0  UpdateFromCAD=off  NumSAPorts=0  CutJoint=off  MarkAsCut=off  Primitives=spherical  PrimitiveProps=S$WORLD$[0 0 0]$spherical  DialogClass=JointBlock  SAxis=[0 0 0]
      settings: SourceProductName=Simscape Multibody  SourceProductBaseCode=MS
  Universal : mblibv1/Joints/Universal  LConnTagsString=__newl0  RConnTagsString=__newr0  UpdateFromCAD=off  NumSAPorts=0  CutJoint=off  MarkAsCut=off  Primitives=prismatic  PrimitiveProps=R1$World$u_axis1$revolute#R2$World$u_axis2$revolute  DialogClass=JointBlock  R1Axis=u_axis1  R2Axis=u_axis2
      settings: SourceProductName=Simscape Multibody  SourceProductBaseCode=MS
  Vector Concatenate : Concatenate  NumInputs=3
  End effector port : PMIOPort  Port=1  Side=Right
  Sphere port : PMIOPort  Port=2  Side=Left
  State : Outport
  wires:
  Joint Sensor/1 -> State/1
  Vector Concatenate/1 -> Joint Actuator/1
  Reaction/1 -> Integrator/1, Vector Concatenate/3
  Integrator/1 -> Integrator1/1, Vector Concatenate/2
  Integrator1/1 -> Vector Concatenate/1
  connections:
  Revolute/RConn1 -- End effector port/RConn1
  Joint Actuator/RConn1 -- Mechanical Branching Bar/RConn1
  Chain RU/RConn1 -- Revolute/LConn1
  Mechanical Branching Bar/LConn1 -- Revolute/LConn2
  Joint Sensor/LConn1 -- Mechanical Branching Bar/RConn2
  Spherical/RConn1 -- Chain US/LConn1
  Universal/RConn1 -- Chain RU/LConn1
  Chain US/RConn1 -- Universal/LConn1
  Sphere port/RConn1 -- Spherical/LConn1
